simulink model "motor_control"  (R2017a)
settings: Solver=VariableStepAuto  StartTime=0.0  StopTime=100  RelTol=1e-3
values from neighbouring files (symbols this model uses):
  I0_1 = 0.0884    [initialization.m]
  In_1 = 4.58    [initialization.m]
  Ki_1 = 0.0934    [initialization.m]
  Ki_re50 = 100*Re50.resistance    [Re50_parameters.m]    (also in Re65_parameters.m = 100*Re65.resistance; initialization.m = 60.8)
  Kp_re50 = 100*Re50.inductance    [Re50_parameters.m]    (also in Re65_parameters.m = 100*Re65.inductance; initialization.m = 42.3)
  Kv_1 = 102*2*pi/60    (= 10.6814150222)    [initialization.m]
  L_1 = 0.423    [initialization.m]
  R_1 = 0.608    [initialization.m]
  V_limit = 45    [initialization.m]
settings Model: Creator=FF  LastModifiedBy=FF

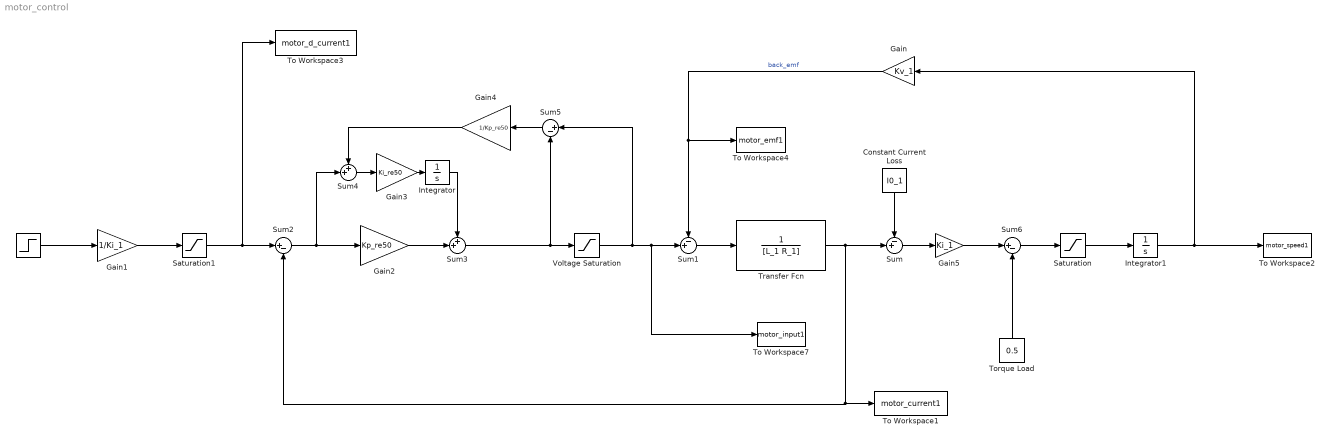
== system motor_control ==
  " " : Step  Time=10  SampleTime=0
  Constant Current Loss : Constant  Value=I0_1
  Gain : Gain  Gain=Kv_1
  Gain1 : Gain  Gain=1/Ki_1
  Gain2 : Gain  Gain=Kp_re50
  Gain3 : Gain  Gain=Ki_re50
  Gain4 : Gain  Gain=1/Kp_re50
  Gain5 : Gain  Gain=Ki_1
  Integrator : Integrator
  Integrator1 : Integrator
  Saturation : Saturate  UpperLimit=10  LowerLimit=0
  Saturation1 : Saturate  UpperLimit=In_1*2  LowerLimit=0
  Sum : Sum  Inputs=-+|
  Sum1 : Sum  Inputs=-+|
  Sum2 : Sum  Inputs=|+-
  Sum3 : Sum  Inputs=++|
  Sum4 : Sum  Inputs=++|
  Sum5 : Sum  Inputs=|+-
  Sum6 : Sum  Inputs=|+-
  To Workspace1 : ToWorkspace  VariableName=motor_current1  SampleTime=-1
  To Workspace2 : ToWorkspace  VariableName=motor_speed1  SampleTime=-1
  To Workspace3 : ToWorkspace  VariableName=motor_d_current1  SampleTime=-1
  To Workspace4 : ToWorkspace  VariableName=motor_emf1  SampleTime=-1
  To Workspace7 : ToWorkspace  VariableName=motor_input1  SampleTime=-1
  Torque Load : Constant  Value=0.5
  Transfer Fcn : TransferFcn  Denominator=[L_1 R_1]
  Voltage Saturation : Saturate  UpperLimit=V_limit  LowerLimit=0
  wires:
  Gain4/1 -> Sum4/1
  Sum5/1 -> Gain4/1
  Integrator/1 -> Sum3/1
  Sum3/1 -> Voltage Saturation/1, Sum5/2
  Gain2/1 -> Sum3/2
  Sum2/1 -> Sum4/2, Gain2/1
  Voltage Saturation/1 -> To Workspace7/1, Sum1/2, Sum5/1
  Gain1/1 -> Saturation1/1
  Gain/1 -> Sum1/1, To Workspace4/1  "back_emf"
  Sum/1 -> Gain5/1
  Sum1/1 -> Transfer Fcn/1
  Constant Current Loss/1 -> Sum/1
  Transfer Fcn/1 -> Sum/2, Sum2/2, To Workspace1/1
  Integrator1/1 -> To Workspace2/1, Gain/1
  Gain3/1 -> Integrator/1
  Sum4/1 -> Gain3/1
  Sum6/1 -> Saturation/1
  Gain5/1 -> Sum6/1
  Torque Load/1 -> Sum6/2
  " "/1 -> Gain1/1
  Saturation/1 -> Integrator1/1
  Saturation1/1 -> To Workspace3/1, Sum2/1
